simulink model "fsproje"  (R2023a)
settings: Solver=daessc  StartTime=0.0  StopTime=100  MaxStep=1e-2  RelTol=1e-3
values from neighbouring files (symbols this model uses):
  b = [0.01 1]    [tfsstwo.m]
  Kd = Kd + 10    (= 20)    [bessaniye.m]    (also in tfss.m = 0.25)
  Ki = 0    [bessaniye.m]    (also in tfss.m = 500)
  Kp = 100    [bessaniye.m]    (also in tfss.m = 21)
undefined symbols (not defined in the file or in its folder): B1, B2, J, J1, J2, K, K1, L, R
libraries: slpidlib x9
(part 1 of 2)
settings Model: Creator=monster  LastModifiedBy=monster
settings SolverCC: MaxConsecutiveMinStep=100000
settings DebuggingCC: MaskedZcDiagnostic=none  IgnoredZcDiagnostic=none

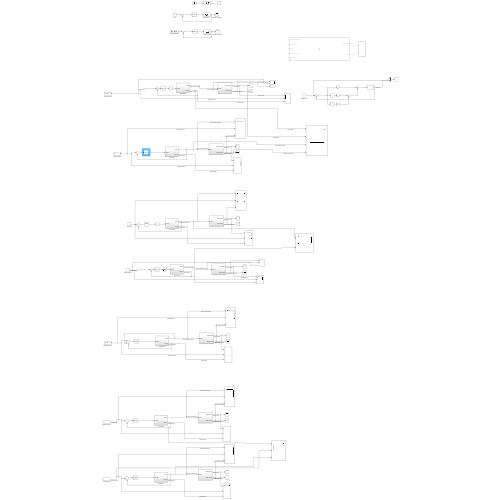
[thumbnail: Simulink's stored preview of the top-level diagram]
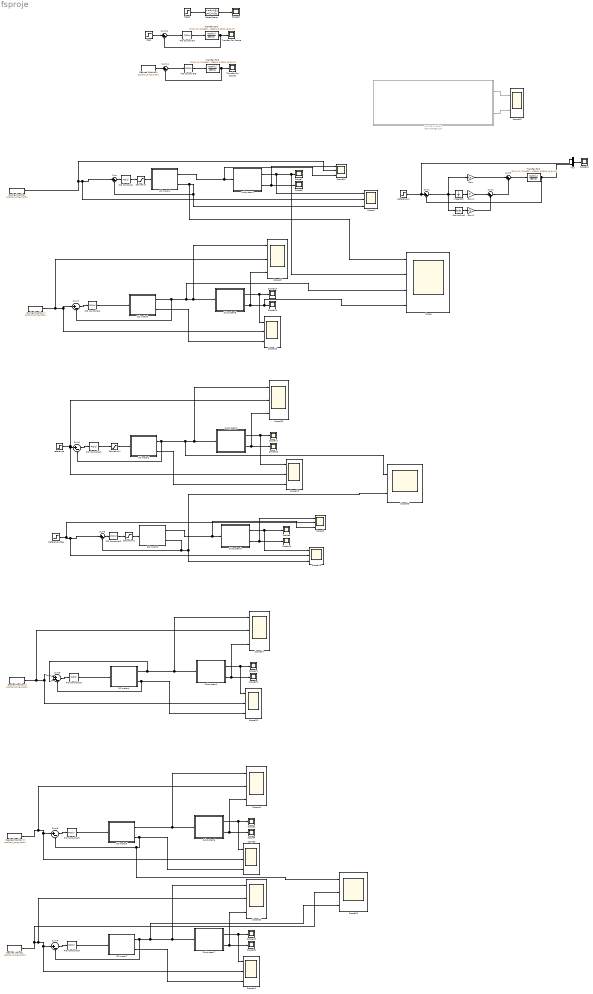
== system fsproje ==
  DC motor1 : Subsystem
  DC motor2 : Subsystem
  DC motor3 : Subsystem
  DC motor4 : Subsystem
  DC motor5 : Subsystem
  DC motor6 : Subsystem
  DC motor7 : Subsystem
  Derivative2 : Derivative
  Desired Position : FromWorkspace  VariableName=position_time_matrix
  Desired Position 1 : FromWorkspace  VariableName=position_time_matrix
  Desired Position 2 : FromWorkspace  VariableName=position_time_matrix
  Desired Position 3 : FromWorkspace  VariableName=position_time_matrix
  Desired Position1 : FromWorkspace  VariableName=position_time_matrix
  Desired Velocity : FromWorkspace  VariableName=position_time_matrix
  Gain : Gain  Gain=Kp
  Gain1 : Gain  Gain=Ki
  Gain2 : Gain  Gain=Kd
  Integrator : Integrator
  MATLAB Function : MATLAB Function  Commented=on  TreatAsAtomicUnit=on
  Mux : Mux  Inputs=2
  PID Controller : slpidlib/PID Controller  Controller=PID  Form=Parallel  TimeDomain=Continuous-time  UseExternalTs=off  SampleTime=-1  IntegratorMethod=Forward Euler  FilterMethod=Forward Euler  ControllerParametersSource=internal  P=58.5763414856901  I=21.7787994337213  UseKiTs=off  D=31.2977676191669  N=613.741127750797  UseFilter=on  TunerSelectOption=Transfer Function Based (PID Tuner App)  InitialConditionSource=internal  InitialConditionForIntegrator=0  InitialConditionForFilter=0  DifferentiatorICPrevScaledInput=0  ExternalReset=none  TrackingMode=off  Kt=1  LimitOutput=off  SatLimitsSource=internal  UpperSaturationLimit=10  LowerSaturationLimit=-10  LinearizeAsGain=on  AntiWindupMode=none  Kb=1  LimitIntegrator=off  UpperIntegratorSaturationLimit=10  LowerIntegratorSaturationLimit=-10  POutMin=[]  POutMax=[]  IOutMin=[]  IOutMax=[]  DOutMin=[]  DOutMax=[]  NOutMin=[]  NOutMax=[]  SumOutMin=[]  SumOutMax=[]  SaturationOutMin=[]  SaturationOutMax=[]  PParamMin=[]  PParamMax=[]  IParamMin=[]  IParamMax=[]  DParamMin=[]  DParamMax=[]  NParamMin=[]  NParamMax=[]  KbParamMin=[]  KbParamMax=[]  KtParamMin=[]  KtParamMax=[]  KbOutMin=[]  KbOutMax=[]  KtOutMin=[]  KtOutMax=[]  IntegratorOutMin=[]  IntegratorOutMax=[]  FilterOutMin=[]  FilterOutMax=[]  SumI1OutMin=[]  SumI1OutMax=[]  SumI2OutMin=[]  SumI2OutMax=[]  SumI3OutMin=[]  SumI3OutMax=[]  SumI4OutMin=[]  SumI4OutMax=[]  SumDOutMin=[]  SumDOutMax=[]  DifferentiatorOutMin=[]  DifferentiatorOutMax=[]  FilterDiffOutCoefMin=[]  FilterDiffOutCoefMax=[]  ReciprocalOutMin=[]  ReciprocalOutMax=[]  SumDenOutMin=[]  SumDenOutMax=[]  SumNumOutMin=[]  SumNumOutMax=[]  DivideOutMin=[]  DivideOutMax=[]  UdiffTsProdOutMin=[]  UdiffTsProdOutMax=[]  NTsProdOutMin=[]  NTsProdOutMax=[]  UintegralTsProdOutMin=[]  UintegralTsProdOutMax=[]  UngainTsProdOutMin=[]  UngainTsProdOutMax=[]  ClampingZeroOutDataTypeStr=Inherit: Inherit via back propagation  ClampingZeroOutMin=[]  ClampingZeroOutMax=[]  FilterDenConstantOutDataTypeStr=Inherit: Inherit via back propagation  FilterDenConstantOutMin=[]  FilterDenConstantOutMax=[]  PCopyOutDataTypeStr=Inherit: Inherit via back propagation  PCopyOutMin=[]  PCopyOutMax=[]  NCopyOutDataTypeStr=Inherit: Inherit via back propagation  NCopyOutMin=[]  NCopyOutMax=[]  IntegratorContinuousStateAttributes=''  IntegratorStateMustResolveToSignalObject=off  IntegratorRTWStateStorageClass=Auto  FilterContinuousStateAttributes=''  FilterStateMustResolveToSignalObject=off  FilterRTWStateStorageClass=Auto  ParallelPVariant=InternalParameters  IdealPVariant=Disabled  IVariant=InternalParameters  DVariant=InternalParameters  IntegratorVariant=Continuous  SatVariant=Disabled  AWVariant=Passthrough  PCopyVariant=Disabled  TRVariant=Disabled  FdbkBlocksVariant=Forward  IdealPFdbkVariant=Disabled  SatFdbkVariant=Disabled  DerivativeFilterVariant=ContFilter  NVariant=InternalParameters  NCopyVariant=Disabled  FilterICVariant=InternalICsFilter  IntegratorICVariant=InternalICs  ExternalResetVariant=Disabled  TRSumVariant=Passthrough  SumFdbkVariant=Disabled  SumVariant=Sum_PID  TsampFilterVariant=InternalTs  TsampNgainVariant=Passthrough  TsampIntegralVariant=Disabled_SignalSpec  ExternalSaturationOutDataTypeStr=Inherit: Same as second input
  PID Controller1 : slpidlib/PID Controller  Controller=PID  Form=Parallel  TimeDomain=Continuous-time  UseExternalTs=off  SampleTime=-1  IntegratorMethod=Forward Euler  FilterMethod=Forward Euler  ControllerParametersSource=internal  P=7.90320095450987  I=25.0422088343632  UseKiTs=off  D=0  N=100  UseFilter=on  TunerSelectOption=Transfer Function Based (PID Tuner App)  InitialConditionSource=internal  InitialConditionForIntegrator=0  InitialConditionForFilter=0  DifferentiatorICPrevScaledInput=0  ExternalReset=none  TrackingMode=off  Kt=1  LimitOutput=off  SatLimitsSource=internal  UpperSaturationLimit=10  LowerSaturationLimit=-10  LinearizeAsGain=on  AntiWindupMode=none  Kb=1  LimitIntegrator=off  UpperIntegratorSaturationLimit=10  LowerIntegratorSaturationLimit=-10  POutMin=[]  POutMax=[]  IOutMin=[]  IOutMax=[]  DOutMin=[]  DOutMax=[]  NOutMin=[]  NOutMax=[]  SumOutMin=[]  SumOutMax=[]  SaturationOutMin=[]  SaturationOutMax=[]  PParamMin=[]  PParamMax=[]  IParamMin=[]  IParamMax=[]  DParamMin=[]  DParamMax=[]  NParamMin=[]  NParamMax=[]  KbParamMin=[]  KbParamMax=[]  KtParamMin=[]  KtParamMax=[]  KbOutMin=[]  KbOutMax=[]  KtOutMin=[]  KtOutMax=[]  IntegratorOutMin=[]  IntegratorOutMax=[]  FilterOutMin=[]  FilterOutMax=[]  SumI1OutMin=[]  SumI1OutMax=[]  SumI2OutMin=[]  SumI2OutMax=[]  SumI3OutMin=[]  SumI3OutMax=[]  SumI4OutMin=[]  SumI4OutMax=[]  SumDOutMin=[]  SumDOutMax=[]  DifferentiatorOutMin=[]  DifferentiatorOutMax=[]  FilterDiffOutCoefMin=[]  FilterDiffOutCoefMax=[]  ReciprocalOutMin=[]  ReciprocalOutMax=[]  SumDenOutMin=[]  SumDenOutMax=[]  SumNumOutMin=[]  SumNumOutMax=[]  DivideOutMin=[]  DivideOutMax=[]  UdiffTsProdOutMin=[]  UdiffTsProdOutMax=[]  NTsProdOutMin=[]  NTsProdOutMax=[]  UintegralTsProdOutMin=[]  UintegralTsProdOutMax=[]  UngainTsProdOutMin=[]  UngainTsProdOutMax=[]  ClampingZeroOutDataTypeStr=Inherit: Inherit via back propagation  ClampingZeroOutMin=[]  ClampingZeroOutMax=[]  FilterDenConstantOutDataTypeStr=Inherit: Inherit via back propagation  FilterDenConstantOutMin=[]  FilterDenConstantOutMax=[]  PCopyOutDataTypeStr=Inherit: Inherit via back propagation  PCopyOutMin=[]  PCopyOutMax=[]  NCopyOutDataTypeStr=Inherit: Inherit via back propagation  NCopyOutMin=[]  NCopyOutMax=[]  IntegratorContinuousStateAttributes=''  IntegratorStateMustResolveToSignalObject=off  IntegratorRTWStateStorageClass=Auto  FilterContinuousStateAttributes=''  FilterStateMustResolveToSignalObject=off  FilterRTWStateStorageClass=Auto  ParallelPVariant=InternalParameters  IdealPVariant=Disabled  IVariant=InternalParameters  DVariant=InternalParameters  IntegratorVariant=Continuous  SatVariant=Disabled  AWVariant=Passthrough  PCopyVariant=Disabled  TRVariant=Disabled  FdbkBlocksVariant=Forward  IdealPFdbkVariant=Disabled  SatFdbkVariant=Disabled  DerivativeFilterVariant=ContFilter  NVariant=InternalParameters  NCopyVariant=Disabled  FilterICVariant=InternalICsFilter  IntegratorICVariant=InternalICs  ExternalResetVariant=Disabled  TRSumVariant=Passthrough  SumFdbkVariant=Disabled  SumVariant=Sum_PID  TsampFilterVariant=InternalTs  TsampNgainVariant=Passthrough  TsampIntegralVariant=Disabled_SignalSpec  ExternalSaturationOutDataTypeStr=Inherit: Same as second input
  PID Controller2 : slpidlib/PID Controller  Controller=PID  Form=Parallel  TimeDomain=Continuous-time  UseExternalTs=off  SampleTime=-1  IntegratorMethod=Forward Euler  FilterMethod=Forward Euler  ControllerParametersSource=internal  P=37.6557555770709  I=10.9348159465012  UseKiTs=off  D=22.0175242854137  N=444.616143119656  UseFilter=on  TunerSelectOption=Transfer Function Based (PID Tuner App)  InitialConditionSource=internal  InitialConditionForIntegrator=0  InitialConditionForFilter=0  DifferentiatorICPrevScaledInput=0  ExternalReset=none  TrackingMode=off  Kt=1  LimitOutput=off  SatLimitsSource=internal  UpperSaturationLimit=10  LowerSaturationLimit=-10  LinearizeAsGain=on  AntiWindupMode=none  Kb=1  LimitIntegrator=off  UpperIntegratorSaturationLimit=10  LowerIntegratorSaturationLimit=-10  POutMin=[]  POutMax=[]  IOutMin=[]  IOutMax=[]  DOutMin=[]  DOutMax=[]  NOutMin=[]  NOutMax=[]  SumOutMin=[]  SumOutMax=[]  SaturationOutMin=[]  SaturationOutMax=[]  PParamMin=[]  PParamMax=[]  IParamMin=[]  IParamMax=[]  DParamMin=[]  DParamMax=[]  NParamMin=[]  NParamMax=[]  KbParamMin=[]  KbParamMax=[]  KtParamMin=[]  KtParamMax=[]  KbOutMin=[]  KbOutMax=[]  KtOutMin=[]  KtOutMax=[]  IntegratorOutMin=[]  IntegratorOutMax=[]  FilterOutMin=[]  FilterOutMax=[]  SumI1OutMin=[]  SumI1OutMax=[]  SumI2OutMin=[]  SumI2OutMax=[]  SumI3OutMin=[]  SumI3OutMax=[]  SumI4OutMin=[]  SumI4OutMax=[]  SumDOutMin=[]  SumDOutMax=[]  DifferentiatorOutMin=[]  DifferentiatorOutMax=[]  FilterDiffOutCoefMin=[]  FilterDiffOutCoefMax=[]  ReciprocalOutMin=[]  ReciprocalOutMax=[]  SumDenOutMin=[]  SumDenOutMax=[]  SumNumOutMin=[]  SumNumOutMax=[]  DivideOutMin=[]  DivideOutMax=[]  UdiffTsProdOutMin=[]  UdiffTsProdOutMax=[]  NTsProdOutMin=[]  NTsProdOutMax=[]  UintegralTsProdOutMin=[]  UintegralTsProdOutMax=[]  UngainTsProdOutMin=[]  UngainTsProdOutMax=[]  ClampingZeroOutDataTypeStr=Inherit: Inherit via back propagation  ClampingZeroOutMin=[]  ClampingZeroOutMax=[]  FilterDenConstantOutDataTypeStr=Inherit: Inherit via back propagation  FilterDenConstantOutMin=[]  FilterDenConstantOutMax=[]  PCopyOutDataTypeStr=Inherit: Inherit via back propagation  PCopyOutMin=[]  PCopyOutMax=[]  NCopyOutDataTypeStr=Inherit: Inherit via back propagation  NCopyOutMin=[]  NCopyOutMax=[]  IntegratorContinuousStateAttributes=''  IntegratorStateMustResolveToSignalObject=off  IntegratorRTWStateStorageClass=Auto  FilterContinuousStateAttributes=''  FilterStateMustResolveToSignalObject=off  FilterRTWStateStorageClass=Auto  ParallelPVariant=InternalParameters  IdealPVariant=Disabled  IVariant=InternalParameters  DVariant=InternalParameters  IntegratorVariant=Continuous  SatVariant=Disabled  AWVariant=Passthrough  PCopyVariant=Disabled  TRVariant=Disabled  FdbkBlocksVariant=Forward  IdealPFdbkVariant=Disabled  SatFdbkVariant=Disabled  DerivativeFilterVariant=ContFilter  NVariant=InternalParameters  NCopyVariant=Disabled  FilterICVariant=InternalICsFilter  IntegratorICVariant=InternalICs  ExternalResetVariant=Disabled  TRSumVariant=Passthrough  SumFdbkVariant=Disabled  SumVariant=Sum_PID  TsampFilterVariant=InternalTs  TsampNgainVariant=Passthrough  TsampIntegralVariant=Disabled_SignalSpec  ExternalSaturationOutDataTypeStr=Inherit: Same as second input
  PID Controller3 : slpidlib/PID Controller  Controller=PID  Form=Parallel  TimeDomain=Continuous-time  UseExternalTs=off  SampleTime=-1  IntegratorMethod=Forward Euler  FilterMethod=Forward Euler  ControllerParametersSource=internal  P=2045.61485829821  I=4710.89336025682  UseKiTs=off  D=197.362863240612  N=45112.732739996  UseFilter=on  TunerSelectOption=Transfer Function Based (PID Tuner App)  InitialConditionSource=internal  InitialConditionForIntegrator=0  InitialConditionForFilter=0  DifferentiatorICPrevScaledInput=0  ExternalReset=none  TrackingMode=off  Kt=1  LimitOutput=off  SatLimitsSource=internal  UpperSaturationLimit=10  LowerSaturationLimit=-10  LinearizeAsGain=on  AntiWindupMode=none  Kb=1  LimitIntegrator=off  UpperIntegratorSaturationLimit=10  LowerIntegratorSaturationLimit=-10  POutMin=[]  POutMax=[]  IOutMin=[]  IOutMax=[]  DOutMin=[]  DOutMax=[]  NOutMin=[]  NOutMax=[]  SumOutMin=[]  SumOutMax=[]  SaturationOutMin=[]  SaturationOutMax=[]  PParamMin=[]  PParamMax=[]  IParamMin=[]  IParamMax=[]  DParamMin=[]  DParamMax=[]  NParamMin=[]  NParamMax=[]  KbParamMin=[]  KbParamMax=[]  KtParamMin=[]  KtParamMax=[]  KbOutMin=[]  KbOutMax=[]  KtOutMin=[]  KtOutMax=[]  IntegratorOutMin=[]  IntegratorOutMax=[]  FilterOutMin=[]  FilterOutMax=[]  SumI1OutMin=[]  SumI1OutMax=[]  SumI2OutMin=[]  SumI2OutMax=[]  SumI3OutMin=[]  SumI3OutMax=[]  SumI4OutMin=[]  SumI4OutMax=[]  SumDOutMin=[]  SumDOutMax=[]  DifferentiatorOutMin=[]  DifferentiatorOutMax=[]  FilterDiffOutCoefMin=[]  FilterDiffOutCoefMax=[]  ReciprocalOutMin=[]  ReciprocalOutMax=[]  SumDenOutMin=[]  SumDenOutMax=[]  SumNumOutMin=[]  SumNumOutMax=[]  DivideOutMin=[]  DivideOutMax=[]  UdiffTsProdOutMin=[]  UdiffTsProdOutMax=[]  NTsProdOutMin=[]  NTsProdOutMax=[]  UintegralTsProdOutMin=[]  UintegralTsProdOutMax=[]  UngainTsProdOutMin=[]  UngainTsProdOutMax=[]  ClampingZeroOutDataTypeStr=Inherit: Inherit via back propagation  ClampingZeroOutMin=[]  ClampingZeroOutMax=[]  FilterDenConstantOutDataTypeStr=Inherit: Inherit via back propagation  FilterDenConstantOutMin=[]  FilterDenConstantOutMax=[]  PCopyOutDataTypeStr=Inherit: Inherit via back propagation  PCopyOutMin=[]  PCopyOutMax=[]  NCopyOutDataTypeStr=Inherit: Inherit via back propagation  NCopyOutMin=[]  NCopyOutMax=[]  IntegratorContinuousStateAttributes=''  IntegratorStateMustResolveToSignalObject=off  IntegratorRTWStateStorageClass=Auto  FilterContinuousStateAttributes=''  FilterStateMustResolveToSignalObject=off  FilterRTWStateStorageClass=Auto  ParallelPVariant=InternalParameters  IdealPVariant=Disabled  IVariant=InternalParameters  DVariant=InternalParameters  IntegratorVariant=Continuous  SatVariant=Disabled  AWVariant=Passthrough  PCopyVariant=Disabled  TRVariant=Disabled  FdbkBlocksVariant=Forward  IdealPFdbkVariant=Disabled  SatFdbkVariant=Disabled  DerivativeFilterVariant=ContFilter  NVariant=InternalParameters  NCopyVariant=Disabled  FilterICVariant=InternalICsFilter  IntegratorICVariant=InternalICs  ExternalResetVariant=Disabled  TRSumVariant=Passthrough  SumFdbkVariant=Disabled  SumVariant=Sum_PID  TsampFilterVariant=InternalTs  TsampNgainVariant=Passthrough  TsampIntegralVariant=Disabled_SignalSpec  ExternalSaturationOutDataTypeStr=Inherit: Same as second input
  PID Controller4 : slpidlib/PID Controller  Controller=PID  Form=Parallel  TimeDomain=Continuous-time  UseExternalTs=off  SampleTime=-1  IntegratorMethod=Forward Euler  FilterMethod=Forward Euler  ControllerParametersSource=internal  P=207.324508460429  I=588.794544524933  UseKiTs=off  D=17.9277897178062  N=4054.94741877744  UseFilter=on  TunerSelectOption=Transfer Function Based (PID Tuner App)  InitialConditionSource=internal  InitialConditionForIntegrator=0  InitialConditionForFilter=0  DifferentiatorICPrevScaledInput=0  ExternalReset=none  TrackingMode=off  Kt=1  LimitOutput=off  SatLimitsSource=internal  UpperSaturationLimit=10  LowerSaturationLimit=-10  LinearizeAsGain=on  AntiWindupMode=none  Kb=1  LimitIntegrator=off  UpperIntegratorSaturationLimit=10  LowerIntegratorSaturationLimit=-10  POutMin=[]  POutMax=[]  IOutMin=[]  IOutMax=[]  DOutMin=[]  DOutMax=[]  NOutMin=[]  NOutMax=[]  SumOutMin=[]  SumOutMax=[]  SaturationOutMin=[]  SaturationOutMax=[]  PParamMin=[]  PParamMax=[]  IParamMin=[]  IParamMax=[]  DParamMin=[]  DParamMax=[]  NParamMin=[]  NParamMax=[]  KbParamMin=[]  KbParamMax=[]  KtParamMin=[]  KtParamMax=[]  KbOutMin=[]  KbOutMax=[]  KtOutMin=[]  KtOutMax=[]  IntegratorOutMin=[]  IntegratorOutMax=[]  FilterOutMin=[]  FilterOutMax=[]  SumI1OutMin=[]  SumI1OutMax=[]  SumI2OutMin=[]  SumI2OutMax=[]  SumI3OutMin=[]  SumI3OutMax=[]  SumI4OutMin=[]  SumI4OutMax=[]  SumDOutMin=[]  SumDOutMax=[]  DifferentiatorOutMin=[]  DifferentiatorOutMax=[]  FilterDiffOutCoefMin=[]  FilterDiffOutCoefMax=[]  ReciprocalOutMin=[]  ReciprocalOutMax=[]  SumDenOutMin=[]  SumDenOutMax=[]  SumNumOutMin=[]  SumNumOutMax=[]  DivideOutMin=[]  DivideOutMax=[]  UdiffTsProdOutMin=[]  UdiffTsProdOutMax=[]  NTsProdOutMin=[]  NTsProdOutMax=[]  UintegralTsProdOutMin=[]  UintegralTsProdOutMax=[]  UngainTsProdOutMin=[]  UngainTsProdOutMax=[]  ClampingZeroOutDataTypeStr=Inherit: Inherit via back propagation  ClampingZeroOutMin=[]  ClampingZeroOutMax=[]  FilterDenConstantOutDataTypeStr=Inherit: Inherit via back propagation  FilterDenConstantOutMin=[]  FilterDenConstantOutMax=[]  PCopyOutDataTypeStr=Inherit: Inherit via back propagation  PCopyOutMin=[]  PCopyOutMax=[]  NCopyOutDataTypeStr=Inherit: Inherit via back propagation  NCopyOutMin=[]  NCopyOutMax=[]  IntegratorContinuousStateAttributes=''  IntegratorStateMustResolveToSignalObject=off  IntegratorRTWStateStorageClass=Auto  FilterContinuousStateAttributes=''  FilterStateMustResolveToSignalObject=off  FilterRTWStateStorageClass=Auto  ParallelPVariant=InternalParameters  IdealPVariant=Disabled  IVariant=InternalParameters  DVariant=InternalParameters  IntegratorVariant=Continuous  SatVariant=Disabled  AWVariant=Passthrough  PCopyVariant=Disabled  TRVariant=Disabled  FdbkBlocksVariant=Forward  IdealPFdbkVariant=Disabled  SatFdbkVariant=Disabled  DerivativeFilterVariant=ContFilter  NVariant=InternalParameters  NCopyVariant=Disabled  FilterICVariant=InternalICsFilter  IntegratorICVariant=InternalICs  ExternalResetVariant=Disabled  TRSumVariant=Passthrough  SumFdbkVariant=Disabled  SumVariant=Sum_PID  TsampFilterVariant=InternalTs  TsampNgainVariant=Passthrough  TsampIntegralVariant=Disabled_SignalSpec  ExternalSaturationOutDataTypeStr=Inherit: Same as second input
  PID Controller5 : slpidlib/PID Controller  Controller=PID  Form=Parallel  TimeDomain=Continuous-time  UseExternalTs=off  SampleTime=-1  IntegratorMethod=Forward Euler  FilterMethod=Forward Euler  ControllerParametersSource=internal  P=55.9637536976089  I=20.0064460537914  UseKiTs=off  D=29.6071796486486  N=586.118226738446  UseFilter=on  TunerSelectOption=Transfer Function Based (PID Tuner App)  InitialConditionSource=internal  InitialConditionForIntegrator=0  InitialConditionForFilter=0  DifferentiatorICPrevScaledInput=0  ExternalReset=none  TrackingMode=off  Kt=1  LimitOutput=off  SatLimitsSource=internal  UpperSaturationLimit=10  LowerSaturationLimit=-10  LinearizeAsGain=on  AntiWindupMode=none  Kb=1  LimitIntegrator=off  UpperIntegratorSaturationLimit=10  LowerIntegratorSaturationLimit=-10  POutMin=[]  POutMax=[]  IOutMin=[]  IOutMax=[]  DOutMin=[]  DOutMax=[]  NOutMin=[]  NOutMax=[]  SumOutMin=[]  SumOutMax=[]  SaturationOutMin=[]  SaturationOutMax=[]  PParamMin=[]  PParamMax=[]  IParamMin=[]  IParamMax=[]  DParamMin=[]  DParamMax=[]  NParamMin=[]  NParamMax=[]  KbParamMin=[]  KbParamMax=[]  KtParamMin=[]  KtParamMax=[]  KbOutMin=[]  KbOutMax=[]  KtOutMin=[]  KtOutMax=[]  IntegratorOutMin=[]  IntegratorOutMax=[]  FilterOutMin=[]  FilterOutMax=[]  SumI1OutMin=[]  SumI1OutMax=[]  SumI2OutMin=[]  SumI2OutMax=[]  SumI3OutMin=[]  SumI3OutMax=[]  SumI4OutMin=[]  SumI4OutMax=[]  SumDOutMin=[]  SumDOutMax=[]  DifferentiatorOutMin=[]  DifferentiatorOutMax=[]  FilterDiffOutCoefMin=[]  FilterDiffOutCoefMax=[]  ReciprocalOutMin=[]  ReciprocalOutMax=[]  SumDenOutMin=[]  SumDenOutMax=[]  SumNumOutMin=[]  SumNumOutMax=[]  DivideOutMin=[]  DivideOutMax=[]  UdiffTsProdOutMin=[]  UdiffTsProdOutMax=[]  NTsProdOutMin=[]  NTsProdOutMax=[]  UintegralTsProdOutMin=[]  UintegralTsProdOutMax=[]  UngainTsProdOutMin=[]  UngainTsProdOutMax=[]  ClampingZeroOutDataTypeStr=Inherit: Inherit via back propagation  ClampingZeroOutMin=[]  ClampingZeroOutMax=[]  FilterDenConstantOutDataTypeStr=Inherit: Inherit via back propagation  FilterDenConstantOutMin=[]  FilterDenConstantOutMax=[]  PCopyOutDataTypeStr=Inherit: Inherit via back propagation  PCopyOutMin=[]  PCopyOutMax=[]  NCopyOutDataTypeStr=Inherit: Inherit via back propagation  NCopyOutMin=[]  NCopyOutMax=[]  IntegratorContinuousStateAttributes=''  IntegratorStateMustResolveToSignalObject=off  IntegratorRTWStateStorageClass=Auto  FilterContinuousStateAttributes=''  FilterStateMustResolveToSignalObject=off  FilterRTWStateStorageClass=Auto  ParallelPVariant=InternalParameters  IdealPVariant=Disabled  IVariant=InternalParameters  DVariant=InternalParameters  IntegratorVariant=Continuous  SatVariant=Disabled  AWVariant=Passthrough  PCopyVariant=Disabled  TRVariant=Disabled  FdbkBlocksVariant=Forward  IdealPFdbkVariant=Disabled  SatFdbkVariant=Disabled  DerivativeFilterVariant=ContFilter  NVariant=InternalParameters  NCopyVariant=Disabled  FilterICVariant=InternalICsFilter  IntegratorICVariant=InternalICs  ExternalResetVariant=Disabled  TRSumVariant=Passthrough  SumFdbkVariant=Disabled  SumVariant=Sum_PID  TsampFilterVariant=InternalTs  TsampNgainVariant=Passthrough  TsampIntegralVariant=Disabled_SignalSpec  ExternalSaturationOutDataTypeStr=Inherit: Same as second input
  PID Controller6 : slpidlib/PID Controller  Controller=PID  Form=Parallel  TimeDomain=Continuous-time  UseExternalTs=off  SampleTime=-1  IntegratorMethod=Forward Euler  FilterMethod=Forward Euler  ControllerParametersSource=internal  P=18.2217269934491  I=51.328469994586  UseKiTs=off  D=0.957542307400605  N=37.219289351236  UseFilter=on  TunerSelectOption=Transfer Function Based (PID Tuner App)  InitialConditionSource=internal  InitialConditionForIntegrator=0  InitialConditionForFilter=0  DifferentiatorICPrevScaledInput=0  ExternalReset=none  TrackingMode=off  Kt=1  LimitOutput=off  SatLimitsSource=internal  UpperSaturationLimit=10  LowerSaturationLimit=-10  LinearizeAsGain=on  AntiWindupMode=none  Kb=1  LimitIntegrator=off  UpperIntegratorSaturationLimit=10  LowerIntegratorSaturationLimit=-10  POutMin=[]  POutMax=[]  IOutMin=[]  IOutMax=[]  DOutMin=[]  DOutMax=[]  NOutMin=[]  NOutMax=[]  SumOutMin=[]  SumOutMax=[]  SaturationOutMin=[]  SaturationOutMax=[]  PParamMin=[]  PParamMax=[]  IParamMin=[]  IParamMax=[]  DParamMin=[]  DParamMax=[]  NParamMin=[]  NParamMax=[]  KbParamMin=[]  KbParamMax=[]  KtParamMin=[]  KtParamMax=[]  KbOutMin=[]  KbOutMax=[]  KtOutMin=[]  KtOutMax=[]  IntegratorOutMin=[]  IntegratorOutMax=[]  FilterOutMin=[]  FilterOutMax=[]  SumI1OutMin=[]  SumI1OutMax=[]  SumI2OutMin=[]  SumI2OutMax=[]  SumI3OutMin=[]  SumI3OutMax=[]  SumI4OutMin=[]  SumI4OutMax=[]  SumDOutMin=[]  SumDOutMax=[]  DifferentiatorOutMin=[]  DifferentiatorOutMax=[]  FilterDiffOutCoefMin=[]  FilterDiffOutCoefMax=[]  ReciprocalOutMin=[]  ReciprocalOutMax=[]  SumDenOutMin=[]  SumDenOutMax=[]  SumNumOutMin=[]  SumNumOutMax=[]  DivideOutMin=[]  DivideOutMax=[]  UdiffTsProdOutMin=[]  UdiffTsProdOutMax=[]  NTsProdOutMin=[]  NTsProdOutMax=[]  UintegralTsProdOutMin=[]  UintegralTsProdOutMax=[]  UngainTsProdOutMin=[]  UngainTsProdOutMax=[]  ClampingZeroOutDataTypeStr=Inherit: Inherit via back propagation  ClampingZeroOutMin=[]  ClampingZeroOutMax=[]  FilterDenConstantOutDataTypeStr=Inherit: Inherit via back propagation  FilterDenConstantOutMin=[]  FilterDenConstantOutMax=[]  PCopyOutDataTypeStr=Inherit: Inherit via back propagation  PCopyOutMin=[]  PCopyOutMax=[]  NCopyOutDataTypeStr=Inherit: Inherit via back propagation  NCopyOutMin=[]  NCopyOutMax=[]  IntegratorContinuousStateAttributes=''  IntegratorStateMustResolveToSignalObject=off  IntegratorRTWStateStorageClass=Auto  FilterContinuousStateAttributes=''  FilterStateMustResolveToSignalObject=off  FilterRTWStateStorageClass=Auto  ParallelPVariant=InternalParameters  IdealPVariant=Disabled  IVariant=InternalParameters  DVariant=InternalParameters  IntegratorVariant=Continuous  SatVariant=Disabled  AWVariant=Passthrough  PCopyVariant=Disabled  TRVariant=Disabled  FdbkBlocksVariant=Forward  IdealPFdbkVariant=Disabled  SatFdbkVariant=Disabled  DerivativeFilterVariant=ContFilter  NVariant=InternalParameters  NCopyVariant=Disabled  FilterICVariant=InternalICsFilter  IntegratorICVariant=InternalICs  ExternalResetVariant=Disabled  TRSumVariant=Passthrough  SumFdbkVariant=Disabled  SumVariant=Sum_PID  TsampFilterVariant=InternalTs  TsampNgainVariant=Passthrough  TsampIntegralVariant=Disabled_SignalSpec  ExternalSaturationOutDataTypeStr=Inherit: Same as second input
  PID Controller7 : slpidlib/PID Controller  Controller=PID  Form=Parallel  TimeDomain=Continuous-time  UseExternalTs=off  SampleTime=-1  IntegratorMethod=Forward Euler  FilterMethod=Forward Euler  ControllerParametersSource=internal  P=40.9250284632695  I=11.6471169726926  UseKiTs=off  D=18.6506512361338  N=402.948949977405  UseFilter=on  TunerSelectOption=Transfer Function Based (PID Tuner App)  InitialConditionSource=internal  InitialConditionForIntegrator=0  InitialConditionForFilter=0  DifferentiatorICPrevScaledInput=0  ExternalReset=none  TrackingMode=off  Kt=1  LimitOutput=off  SatLimitsSource=internal  UpperSaturationLimit=inf  LowerSaturationLimit=-inf  LinearizeAsGain=on  AntiWindupMode=none  Kb=1  LimitIntegrator=off  UpperIntegratorSaturationLimit=inf  LowerIntegratorSaturationLimit=-inf  POutMin=[]  POutMax=[]  IOutMin=[]  IOutMax=[]  DOutMin=[]  DOutMax=[]  NOutMin=[]  NOutMax=[]  SumOutMin=[]  SumOutMax=[]  SaturationOutMin=[]  SaturationOutMax=[]  PParamMin=[]  PParamMax=[]  IParamMin=[]  IParamMax=[]  DParamMin=[]  DParamMax=[]  NParamMin=[]  NParamMax=[]  KbParamMin=[]  KbParamMax=[]  KtParamMin=[]  KtParamMax=[]  KbOutMin=[]  KbOutMax=[]  KtOutMin=[]  KtOutMax=[]  IntegratorOutMin=[]  IntegratorOutMax=[]  FilterOutMin=[]  FilterOutMax=[]  SumI1OutMin=[]  SumI1OutMax=[]  SumI2OutMin=[]  SumI2OutMax=[]  SumI3OutMin=[]  SumI3OutMax=[]  SumI4OutMin=[]  SumI4OutMax=[]  SumDOutMin=[]  SumDOutMax=[]  DifferentiatorOutMin=[]  DifferentiatorOutMax=[]  FilterDiffOutCoefMin=[]  FilterDiffOutCoefMax=[]  ReciprocalOutMin=[]  ReciprocalOutMax=[]  SumDenOutMin=[]  SumDenOutMax=[]  SumNumOutMin=[]  SumNumOutMax=[]  DivideOutMin=[]  DivideOutMax=[]  UdiffTsProdOutMin=[]  UdiffTsProdOutMax=[]  NTsProdOutMin=[]  NTsProdOutMax=[]  UintegralTsProdOutMin=[]  UintegralTsProdOutMax=[]  UngainTsProdOutMin=[]  UngainTsProdOutMax=[]  ClampingZeroOutDataTypeStr=Inherit: Inherit via back propagation  ClampingZeroOutMin=[]  ClampingZeroOutMax=[]  FilterDenConstantOutDataTypeStr=Inherit: Inherit via back propagation  FilterDenConstantOutMin=[]  FilterDenConstantOutMax=[]  PCopyOutDataTypeStr=Inherit: Inherit via back propagation  PCopyOutMin=[]  PCopyOutMax=[]  NCopyOutDataTypeStr=Inherit: Inherit via back propagation  NCopyOutMin=[]  NCopyOutMax=[]  IntegratorContinuousStateAttributes=''  IntegratorStateMustResolveToSignalObject=off  IntegratorRTWStateStorageClass=Auto  FilterContinuousStateAttributes=''  FilterStateMustResolveToSignalObject=off  FilterRTWStateStorageClass=Auto  ParallelPVariant=InternalParameters  IdealPVariant=Disabled  IVariant=InternalParameters  DVariant=InternalParameters  IntegratorVariant=Continuous  SatVariant=Disabled  AWVariant=Passthrough  PCopyVariant=Disabled  TRVariant=Disabled  FdbkBlocksVariant=Forward  IdealPFdbkVariant=Disabled  SatFdbkVariant=Disabled  DerivativeFilterVariant=ContFilter  NVariant=InternalParameters  NCopyVariant=Disabled  FilterICVariant=InternalICsFilter  IntegratorICVariant=InternalICs  ExternalResetVariant=Disabled  TRSumVariant=Passthrough  SumFdbkVariant=Disabled  SumVariant=Sum_PID  TsampFilterVariant=InternalTs  TsampNgainVariant=Passthrough  TsampIntegralVariant=Disabled_SignalSpec  ExternalSaturationOutDataTypeStr=Inherit: Same as second input
  PID Controller8 : slpidlib/PID Controller  Controller=PID  Form=Parallel  TimeDomain=Continuous-time  UseExternalTs=off  SampleTime=-1  IntegratorMethod=Forward Euler  FilterMethod=Forward Euler  ControllerParametersSource=internal  P=40.9250284632695  I=11.6471169726926  UseKiTs=off  D=18.6506512361338  N=402.948949977405  UseFilter=on  TunerSelectOption=Transfer Function Based (PID Tuner App)  InitialConditionSource=internal  InitialConditionForIntegrator=0  InitialConditionForFilter=0  DifferentiatorICPrevScaledInput=0  ExternalReset=none  TrackingMode=off  Kt=1  LimitOutput=off  SatLimitsSource=internal  UpperSaturationLimit=inf  LowerSaturationLimit=-inf  LinearizeAsGain=on  AntiWindupMode=none  Kb=1  LimitIntegrator=off  UpperIntegratorSaturationLimit=inf  LowerIntegratorSaturationLimit=-inf  POutMin=[]  POutMax=[]  IOutMin=[]  IOutMax=[]  DOutMin=[]  DOutMax=[]  NOutMin=[]  NOutMax=[]  SumOutMin=[]  SumOutMax=[]  SaturationOutMin=[]  SaturationOutMax=[]  PParamMin=[]  PParamMax=[]  IParamMin=[]  IParamMax=[]  DParamMin=[]  DParamMax=[]  NParamMin=[]  NParamMax=[]  KbParamMin=[]  KbParamMax=[]  KtParamMin=[]  KtParamMax=[]  KbOutMin=[]  KbOutMax=[]  KtOutMin=[]  KtOutMax=[]  IntegratorOutMin=[]  IntegratorOutMax=[]  FilterOutMin=[]  FilterOutMax=[]  SumI1OutMin=[]  SumI1OutMax=[]  SumI2OutMin=[]  SumI2OutMax=[]  SumI3OutMin=[]  SumI3OutMax=[]  SumI4OutMin=[]  SumI4OutMax=[]  SumDOutMin=[]  SumDOutMax=[]  DifferentiatorOutMin=[]  DifferentiatorOutMax=[]  FilterDiffOutCoefMin=[]  FilterDiffOutCoefMax=[]  ReciprocalOutMin=[]  ReciprocalOutMax=[]  SumDenOutMin=[]  SumDenOutMax=[]  SumNumOutMin=[]  SumNumOutMax=[]  DivideOutMin=[]  DivideOutMax=[]  UdiffTsProdOutMin=[]  UdiffTsProdOutMax=[]  NTsProdOutMin=[]  NTsProdOutMax=[]  UintegralTsProdOutMin=[]  UintegralTsProdOutMax=[]  UngainTsProdOutMin=[]  UngainTsProdOutMax=[]  ClampingZeroOutDataTypeStr=Inherit: Inherit via back propagation  ClampingZeroOutMin=[]  ClampingZeroOutMax=[]  FilterDenConstantOutDataTypeStr=Inherit: Inherit via back propagation  FilterDenConstantOutMin=[]  FilterDenConstantOutMax=[]  PCopyOutDataTypeStr=Inherit: Inherit via back propagation  PCopyOutMin=[]  PCopyOutMax=[]  NCopyOutDataTypeStr=Inherit: Inherit via back propagation  NCopyOutMin=[]  NCopyOutMax=[]  IntegratorContinuousStateAttributes=''  IntegratorStateMustResolveToSignalObject=off  IntegratorRTWStateStorageClass=Auto  FilterContinuousStateAttributes=''  FilterStateMustResolveToSignalObject=off  FilterRTWStateStorageClass=Auto  ParallelPVariant=InternalParameters  IdealPVariant=Disabled  IVariant=InternalParameters  DVariant=InternalParameters  IntegratorVariant=Continuous  SatVariant=Disabled  AWVariant=Passthrough  PCopyVariant=Disabled  TRVariant=Disabled  FdbkBlocksVariant=Forward  IdealPFdbkVariant=Disabled  SatFdbkVariant=Disabled  DerivativeFilterVariant=ContFilter  NVariant=InternalParameters  NCopyVariant=Disabled  FilterICVariant=InternalICsFilter  IntegratorICVariant=InternalICs  ExternalResetVariant=Disabled  TRSumVariant=Passthrough  SumFdbkVariant=Disabled  SumVariant=Sum_PID  TsampFilterVariant=InternalTs  TsampNgainVariant=Passthrough  TsampIntegralVariant=Disabled_SignalSpec  ExternalSaturationOutDataTypeStr=Inherit: Same as second input
  Reference 2 : Step  SampleTime=0
  Reference Step : Step  After=5  SampleTime=0
  Saturation : Saturate  UpperLimit=50  LowerLimit=-50
  Saturation1 : Saturate  UpperLimit=100000  LowerLimit=-100000
  Saturation2 : Saturate  UpperLimit=100000  LowerLimit=-100000
  Scope : Scope  NumInputPorts=4
  Scope{1,3,9..10,13..14,19..20,23..24,26..28,31..32} (15 alike) : Scope  NumInputPorts=3
  Scope{2,4..8,11..12,15,17..18,21..22,25,29..30} (16 alike) : Scope
  Scope16 : Scope  NumInputPorts=2
  Scope33 : Scope  NumInputPorts=2
  State-Space : StateSpace  A=[-32 -1260 -12400 -20020 0; 1 0 0 0 0; 0 1 0 0 0; 0 0 1 0 0; 0 0 0 1 0]  B=[1; 0; 0; 0; 0]  C=[0 0 0 20 2000]  D=[0]  InitialCondition=[0;0;0;0;0]
  Step : Step  After=5  SampleTime=0
  Step2 : Step  After=5  SampleTime=0
  Subsystem1 : Subsystem
  Subsystem2 : Subsystem
  Subsystem3 : Subsystem
  Subsystem4 : Subsystem
  Subsystem5 : Subsystem
  Subsystem6 : Subsystem
  Subsystem7 : Subsystem
  Sum{,1,4..5,7..11} (9 alike) : Sum  Inputs=|+-
  Sum2 : Sum  Inputs=|++
  Sum3 : Sum  Inputs=|++
  Sum6 : Sum  Inputs=|+--
  Transfer Fcn Scope : Scope
  Transfer Fcn Scope1 : Scope
  Transfer Fcn1 : TransferFcn  Numerator=[0.01 1]  Denominator=[0.0005 0.016 0.63001 6.2002 10.01 0]
  Transfer Fcn2 : TransferFcn  Numerator=[0.01 1]  Denominator=[0.0005 0.016 0.63001 6.2002 10.01 0]
  Transfer Fcn3 : TransferFcn  Numerator=[0.01 1]  Denominator=[0.0005 0.016 0.63001 6.2002 10.01 0]
  reference : Step  After=5  SampleTime=0
  wires:
  Integrator/1 -> Gain1/1
  DC motor2/1(Speed) -> Scope33/1, Scope20/1, Subsystem2/1(Speed), Sum4/2  "Motor Velocity Simulink"
  Gain1/1 -> Sum2/1
  MATLAB Function/1(position_radian) -> Scope16/1
  reference/1 -> Sum4/1, Scope19/2, Scope20/2
  Sum/1 -> PID Controller/1
  Reference 2/1 -> Mux/1, Sum1/1
  Sum4/1 -> PID Controller1/1
  Subsystem2/2(Shaft Velocity) -> Scope20/3, Scope18/1  "Shaft Velocity Simulink"
  Gain/1 -> Sum3/1
  Transfer Fcn2/1 -> Sum1/2, Mux/2  "Position"
  Subsystem1/2(Shaft Velocity) -> Scope10/1, Scope8/1  "Shaft Velocity Simulink"
  MATLAB Function/2(velocity) -> Scope16/2
  Saturation/1 -> DC motor1/1(voltage)
  Subsystem1/1(Shaft Position) -> Scope1/1, Scope/2, Scope7/1  "Shaft Position"
  Gain2/1 -> Sum2/2
  Sum2/1 -> Sum3/2
  Derivative2/1 -> Gain2/1
  Subsystem2/1(Shaft Position) -> Scope19/1, Scope17/1  "Shaft Position"
  PID Controller/1 -> Saturation/1
  Sum3/1 -> Transfer Fcn2/1
  Sum1/1 -> Derivative2/1, Gain/1, Integrator/1
  DC motor2/2(Position) -> Scope19/3  "Motor Position"
  DC motor1/1(Speed) -> Scope10/3, Subsystem1/1(Speed)  "Motor Velocity Simulink"
  Mux/1 -> Scope12/1
  PID Controller1/1 -> Saturation1/1
  DC motor1/2(Position) -> Scope/1, Scope1/3, Sum/2  "Motor Position"
  State-Space/1 -> Scope5/1
  Step2/1 -> State-Space/1
  Transfer Fcn1/1 -> Transfer Fcn Scope/1, Sum10/2
  Desired Position/1 -> Scope10/2, Scope1/2, Sum/1  "Desired Position"
  Saturation1/1 -> DC motor2/1(voltage)
  Reference Step/1 -> Scope13/2, Sum5/1, Scope3/2  "Reference step"
  DC motor3/2(Position) -> Sum5/2, Scope33/2, Scope13/3  "Motor Position"
  PID Controller2/1 -> Saturation2/1
  DC motor3/1(Speed) -> Scope3/3, Subsystem3/1(Speed)  "Motor Velocity Simulink"
  Subsystem3/1(Shaft Position) -> Scope13/1, Scope6/1  "Shaft Position"
  Subsystem3/2(Shaft Velocity) -> Scope3/1, Scope11/1  "Shaft Velocity Simulink"
  Saturation2/1 -> DC motor3/1(voltage)
  Sum5/1 -> PID Controller2/1
  Subsystem4/2(Shaft Velocity) -> Scope24/3, Scope22/1  "Shaft Velocity Simulink"
  Sum6/1 -> PID Controller3/1
  DC motor4/2(Position) -> Scope23/3, Sum6/3  "Motor Position"
  Subsystem4/1(Shaft Position) -> Scope23/1, Scope21/1  "Shaft Position"
  DC motor4/1(Speed) -> Sum6/2, Scope24/1, Subsystem4/1(Speed)  "Motor Velocity Simulink"
  Desired Position 2/1 -> Scope24/2, Scope23/2, Sum6/1  "Desired Position 2"
  PID Controller3/1 -> DC motor4/1(voltage)
  DC motor5/2(Position) -> Scope26/3  "Motor Position"
  Desired Position 1/1 -> Scope27/2, Scope26/2, Sum7/1  "Desired Position 2"
  PID Controller4/1 -> DC motor5/1(voltage)
  Sum7/1 -> PID Controller4/1
  Subsystem5/2(Shaft Velocity) -> Scope27/3, Scope/4, Scope25/1  "Shaft Velocity Simulink"
  DC motor5/1(Speed) -> Scope/3, Scope27/1, Subsystem5/1(Speed), Sum7/2  "Motor Velocity Simulink"
  Subsystem5/1(Shaft Position) -> Scope26/1, Scope15/1  "Shaft Position"
  PID Controller5/1 -> DC motor6/1(voltage)
  DC motor6/2(Position) -> Scope32/1, Sum8/2, Scope9/3  "Motor Position"
  DC motor6/1(Speed) -> Scope14/1, Subsystem6/1(Speed)  "Motor Velocity Simulink"
  Subsystem6/1(Shaft Position) -> Scope9/1, Scope2/1  "Shaft Position"
  Subsystem6/2(Shaft Velocity) -> Scope14/3, Scope4/1  "Shaft Velocity Simulink"
  Sum8/1 -> PID Controller5/1
  Desired Position 3/1 -> Scope14/2, Scope9/2, Sum8/1  "Desired Position"
  Desired Velocity/1 -> Scope32/2, Sum9/1, Scope31/2, Scope28/2  "Desired Velocity"
  Sum9/1 -> PID Controller6/1
  Subsystem7/2(Shaft Velocity) -> Scope30/1, Scope28/3  "Shaft Velocity Simulink"
  Subsystem7/1(Shaft Position) -> Scope29/1, Scope31/1  "Shaft Position"
  DC motor7/1(Speed) -> Scope32/3, Subsystem7/1(Speed), Scope28/1, Sum9/2  "Motor Velocity Simulink"
  DC motor7/2(Position) -> Scope31/3  "Motor Position"
  PID Controller6/1 -> DC motor7/1(voltage)
  PID Controller7/1 -> Transfer Fcn1/1
  Step/1 -> Sum10/1
  Sum10/1 -> PID Controller7/1
  PID Controller8/1 -> Transfer Fcn3/1
  Transfer Fcn3/1 -> Transfer Fcn Scope1/1, Sum11/2
  Sum11/1 -> PID Controller8/1
  Desired Position1/1 -> Sum11/1

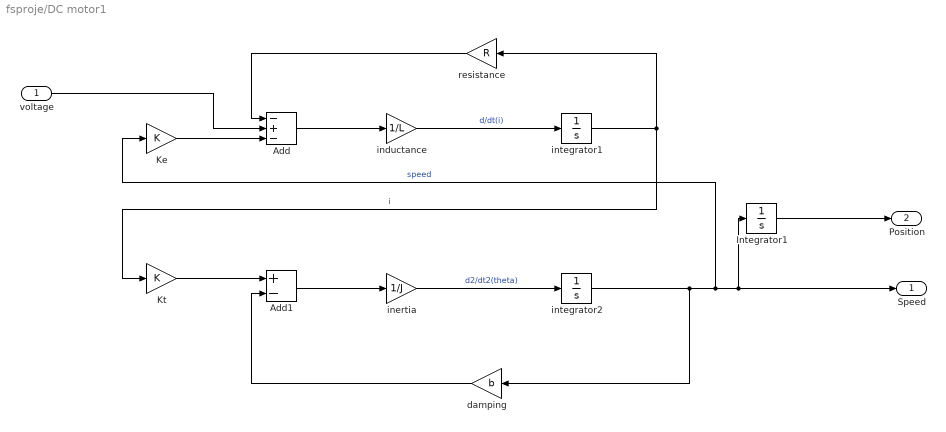
== system fsproje/DC motor1 ==
  voltage : Inport
  Add : Sum  Inputs=-+-
  Add1 : Sum  Inputs=+-
  Integrator1 : Integrator
  Ke : Gain  Gain=K
  Kt : Gain  Gain=K
  damping : Gain  Gain=b
  "inductance " : Gain  Gain=1/L
  inertia : Gain  Gain=1/J
  integrator1 : Integrator
  integrator2 : Integrator
  resistance : Gain  Gain=R
  Speed : Outport
  Position : Outport  Port=2
  wires:
  damping/1 -> Add1/2
  Add1/1 -> inertia/1
  Kt/1 -> Add1/1
  integrator1/1 -> resistance/1, Kt/1  "i"
  Add/1 -> "inductance "/1
  voltage/1 -> Add/2
  resistance/1 -> Add/1
  inertia/1 -> integrator2/1  "d2/dt2(theta)"
  integrator2/1 -> damping/1, Integrator1/1, Speed/1, Ke/1  "speed"
  Ke/1 -> Add/3
  "inductance "/1 -> integrator1/1  "d/dt(i)"
  Integrator1/1 -> Position/1

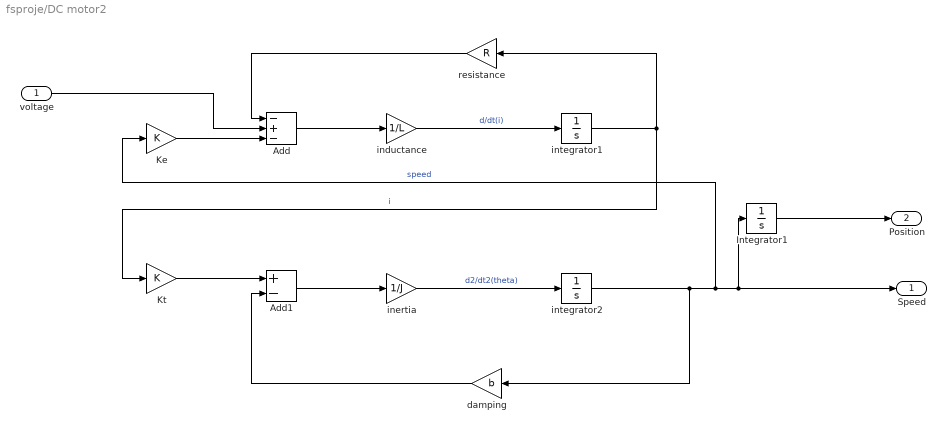
== system fsproje/DC motor2 ==
  voltage : Inport
  Add : Sum  Inputs=-+-
  Add1 : Sum  Inputs=+-
  Integrator1 : Integrator
  Ke : Gain  Gain=K
  Kt : Gain  Gain=K
  damping : Gain  Gain=b
  "inductance " : Gain  Gain=1/L
  inertia : Gain  Gain=1/J
  integrator1 : Integrator
  integrator2 : Integrator
  resistance : Gain  Gain=R
  Speed : Outport
  Position : Outport  Port=2
  wires:
  damping/1 -> Add1/2
  Add1/1 -> inertia/1
  Kt/1 -> Add1/1
  integrator1/1 -> resistance/1, Kt/1  "i"
  Add/1 -> "inductance "/1
  voltage/1 -> Add/2
  resistance/1 -> Add/1
  inertia/1 -> integrator2/1  "d2/dt2(theta)"
  integrator2/1 -> damping/1, Integrator1/1, Speed/1, Ke/1  "speed"
  Ke/1 -> Add/3
  "inductance "/1 -> integrator1/1  "d/dt(i)"
  Integrator1/1 -> Position/1

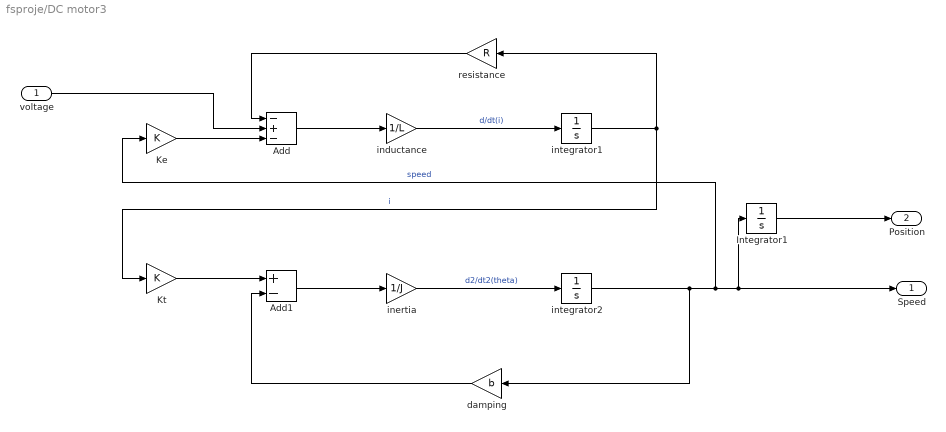
== system fsproje/DC motor3 ==
  voltage : Inport
  Add : Sum  Inputs=-+-
  Add1 : Sum  Inputs=+-
  Integrator1 : Integrator
  Ke : Gain  Gain=K
  Kt : Gain  Gain=K
  damping : Gain  Gain=b
  "inductance " : Gain  Gain=1/L
  inertia : Gain  Gain=1/J
  integrator1 : Integrator
  integrator2 : Integrator
  resistance : Gain  Gain=R
  Speed : Outport
  Position : Outport  Port=2
  wires:
  damping/1 -> Add1/2
  Add1/1 -> inertia/1
  Kt/1 -> Add1/1
  integrator1/1 -> resistance/1, Kt/1  "i"
  Add/1 -> "inductance "/1
  voltage/1 -> Add/2
  resistance/1 -> Add/1
  inertia/1 -> integrator2/1  "d2/dt2(theta)"
  integrator2/1 -> damping/1, Integrator1/1, Speed/1, Ke/1  "speed"
  Ke/1 -> Add/3
  "inductance "/1 -> integrator1/1  "d/dt(i)"
  Integrator1/1 -> Position/1

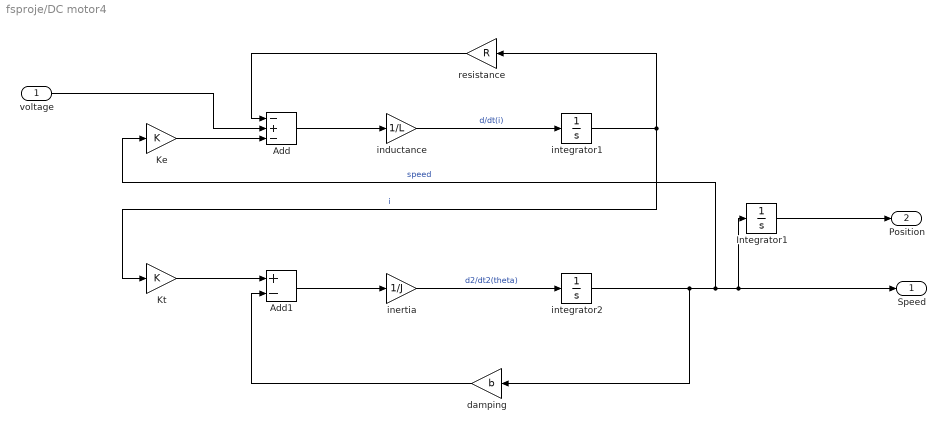
== system fsproje/DC motor4 ==
  voltage : Inport
  Add : Sum  Inputs=-+-
  Add1 : Sum  Inputs=+-
  Integrator1 : Integrator
  Ke : Gain  Gain=K
  Kt : Gain  Gain=K
  damping : Gain  Gain=b
  "inductance " : Gain  Gain=1/L
  inertia : Gain  Gain=1/J
  integrator1 : Integrator
  integrator2 : Integrator
  resistance : Gain  Gain=R
  Speed : Outport
  Position : Outport  Port=2
  wires:
  damping/1 -> Add1/2
  Add1/1 -> inertia/1
  Kt/1 -> Add1/1
  integrator1/1 -> resistance/1, Kt/1  "i"
  Add/1 -> "inductance "/1
  voltage/1 -> Add/2
  resistance/1 -> Add/1
  inertia/1 -> integrator2/1  "d2/dt2(theta)"
  integrator2/1 -> damping/1, Integrator1/1, Speed/1, Ke/1  "speed"
  Ke/1 -> Add/3
  "inductance "/1 -> integrator1/1  "d/dt(i)"
  Integrator1/1 -> Position/1

== system fsproje/DC motor5 ==
  voltage : Inport
  Add : Sum  Inputs=-+-
  Add1 : Sum  Inputs=+-
  Integrator1 : Integrator
  Ke : Gain  Gain=K
  Kt : Gain  Gain=K
  damping : Gain  Gain=b
  "inductance " : Gain  Gain=1/L
  inertia : Gain  Gain=1/J
  integrator1 : Integrator
  integrator2 : Integrator
  resistance : Gain  Gain=R
  Speed : Outport
  Position : Outport  Port=2
  wires:
  damping/1 -> Add1/2
  Add1/1 -> inertia/1
  Kt/1 -> Add1/1
  integrator1/1 -> resistance/1, Kt/1  "i"
  Add/1 -> "inductance "/1
  voltage/1 -> Add/2
  resistance/1 -> Add/1
  inertia/1 -> integrator2/1  "d2/dt2(theta)"
  integrator2/1 -> damping/1, Integrator1/1, Speed/1, Ke/1  "speed"
  Ke/1 -> Add/3
  "inductance "/1 -> integrator1/1  "d/dt(i)"
  Integrator1/1 -> Position/1

== system fsproje/DC motor6 ==
  voltage : Inport
  Add : Sum  Inputs=-+-
  Add1 : Sum  Inputs=+-
  Integrator1 : Integrator
  Ke : Gain  Gain=K
  Kt : Gain  Gain=K
  damping : Gain  Gain=b
  "inductance " : Gain  Gain=1/L
  inertia : Gain  Gain=1/J
  integrator1 : Integrator
  integrator2 : Integrator
  resistance : Gain  Gain=R
  Speed : Outport
  Position : Outport  Port=2
  wires:
  damping/1 -> Add1/2
  Add1/1 -> inertia/1
  Kt/1 -> Add1/1
  integrator1/1 -> resistance/1, Kt/1  "i"
  Add/1 -> "inductance "/1
  voltage/1 -> Add/2
  resistance/1 -> Add/1
  inertia/1 -> integrator2/1  "d2/dt2(theta)"
  integrator2/1 -> damping/1, Integrator1/1, Speed/1, Ke/1  "speed"
  Ke/1 -> Add/3
  "inductance "/1 -> integrator1/1  "d/dt(i)"
  Integrator1/1 -> Position/1

== system fsproje/DC motor7 ==
  voltage : Inport
  Add : Sum  Inputs=-+-
  Add1 : Sum  Inputs=+-
  Integrator1 : Integrator
  Ke : Gain  Gain=K
  Kt : Gain  Gain=K
  damping : Gain  Gain=b
  "inductance " : Gain  Gain=1/L
  inertia : Gain  Gain=1/J
  integrator1 : Integrator
  integrator2 : Integrator
  resistance : Gain  Gain=R
  Speed : Outport
  Position : Outport  Port=2
  wires:
  Integrator1/1 -> Position/1
  "inductance "/1 -> integrator1/1  "d/dt(i)"
  Ke/1 -> Add/3
  integrator2/1 -> Ke/1, Speed/1, Integrator1/1, damping/1  "speed"
  inertia/1 -> integrator2/1  "d2/dt2(theta)"
  resistance/1 -> Add/1
  voltage/1 -> Add/2
  Add/1 -> "inductance "/1
  integrator1/1 -> Kt/1, resistance/1  "i"
  Kt/1 -> Add1/1
  Add1/1 -> inertia/1
  damping/1 -> Add1/2

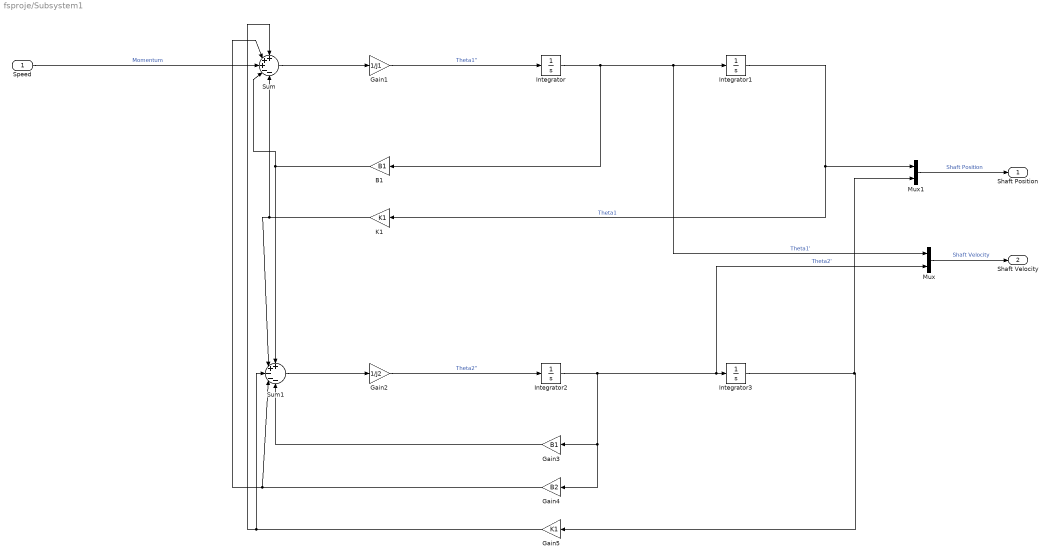
== system fsproje/Subsystem1 ==
  Speed : Inport
  B1 : Gain  Gain=B1
  Gain1 : Gain  Gain=1/J1
  Gain2 : Gain  Gain=1/J2
  Gain3 : Gain  Gain=B1
  Gain4 : Gain  Gain=B2
  Gain5 : Gain  Gain=K1
  Integrator{,1..3} (4 alike) : Integrator
  K1 : Gain  Gain=K1
  Mux : Mux  Inputs=2
  Mux1 : Mux  Inputs=2
  Sum : Sum  Inputs=+++--
  Sum1 : Sum  Inputs=++---
  Shaft Position : Outport
  Shaft Velocity : Outport  Port=2
  wires:
  Gain5/1 -> Sum1/3, Sum/1
  Integrator3/1 -> Gain5/1, Mux1/2
  Gain4/1 -> Sum/2, Sum1/4
  Gain3/1 -> Sum1/5
  Integrator2/1 -> Mux/2, Integrator3/1, Gain3/1, Gain4/1  "Theta2'"
  Gain2/1 -> Integrator2/1  "Theta2''"
  Sum1/1 -> Gain2/1
  K1/1 -> Sum1/2, Sum/5
  Integrator1/1 -> Mux1/1, K1/1  "Theta1"
  B1/1 -> Sum/4, Sum1/1
  Integrator/1 -> Mux/1, Integrator1/1, B1/1  "Theta1'"
  Gain1/1 -> Integrator/1  "Theta1''"
  Speed/1 -> Sum/3  "Momentum"
  Sum/1 -> Gain1/1
  Mux1/1 -> Shaft Position/1  "Shaft Position"
  Mux/1 -> Shaft Velocity/1  "Shaft Velocity"

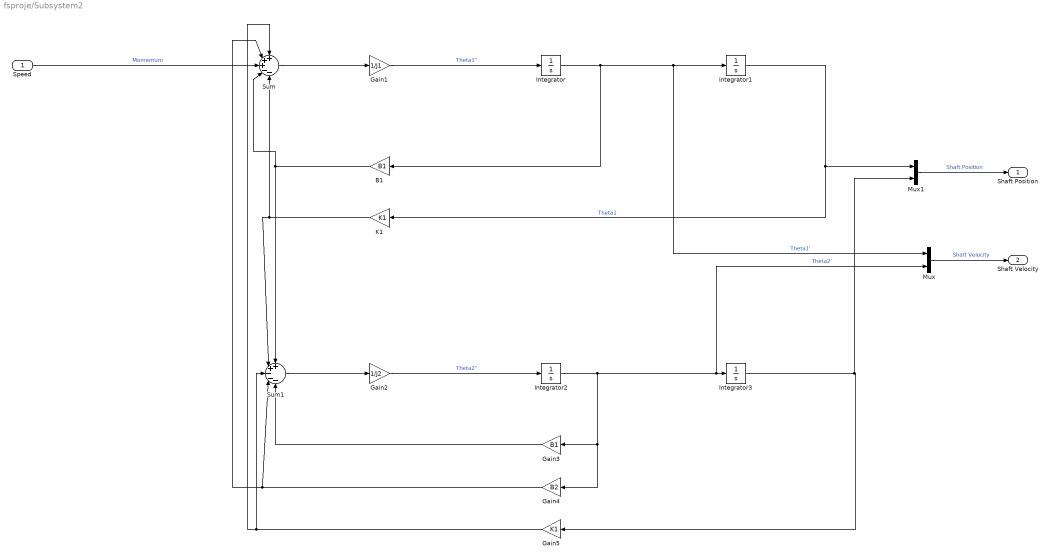
== system fsproje/Subsystem2 ==
  Speed : Inport
  B1 : Gain  Gain=B1
  Gain1 : Gain  Gain=1/J1
  Gain2 : Gain  Gain=1/J2
  Gain3 : Gain  Gain=B1
  Gain4 : Gain  Gain=B2
  Gain5 : Gain  Gain=K1
  Integrator{,1..3} (4 alike) : Integrator
  K1 : Gain  Gain=K1
  Mux : Mux  Inputs=2
  Mux1 : Mux  Inputs=2
  Sum : Sum  Inputs=+++--
  Sum1 : Sum  Inputs=++---
  Shaft Position : Outport
  Shaft Velocity : Outport  Port=2
  wires:
  Gain5/1 -> Sum1/3, Sum/1
  Integrator3/1 -> Gain5/1, Mux1/2
  Gain4/1 -> Sum/2, Sum1/4
  Gain3/1 -> Sum1/5
  Integrator2/1 -> Mux/2, Integrator3/1, Gain3/1, Gain4/1  "Theta2'"
  Gain2/1 -> Integrator2/1  "Theta2''"
  Sum1/1 -> Gain2/1
  K1/1 -> Sum1/2, Sum/5
  Integrator1/1 -> Mux1/1, K1/1  "Theta1"
  B1/1 -> Sum/4, Sum1/1
  Integrator/1 -> Mux/1, Integrator1/1, B1/1  "Theta1'"
  Gain1/1 -> Integrator/1  "Theta1''"
  Speed/1 -> Sum/3  "Momentum"
  Sum/1 -> Gain1/1
  Mux1/1 -> Shaft Position/1  "Shaft Position"
  Mux/1 -> Shaft Velocity/1  "Shaft Velocity"

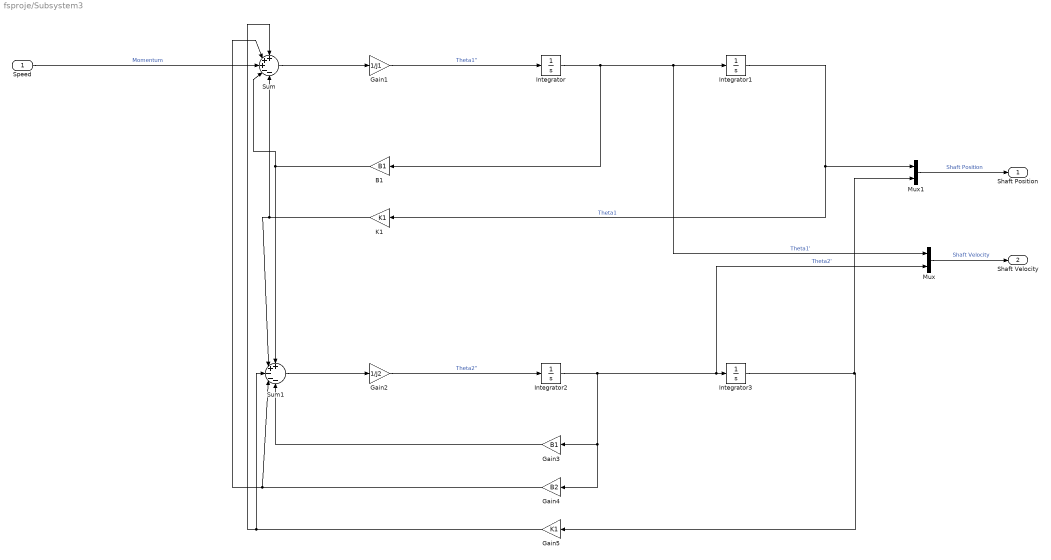
== system fsproje/Subsystem3 ==
  Speed : Inport
  B1 : Gain  Gain=B1
  Gain1 : Gain  Gain=1/J1
  Gain2 : Gain  Gain=1/J2
  Gain3 : Gain  Gain=B1
  Gain4 : Gain  Gain=B2
  Gain5 : Gain  Gain=K1
  Integrator{,1..3} (4 alike) : Integrator
  K1 : Gain  Gain=K1
  Mux : Mux  Inputs=2
  Mux1 : Mux  Inputs=2
  Sum : Sum  Inputs=+++--
  Sum1 : Sum  Inputs=++---
  Shaft Position : Outport
  Shaft Velocity : Outport  Port=2
  wires:
  Gain5/1 -> Sum1/3, Sum/1
  Integrator3/1 -> Gain5/1, Mux1/2
  Gain4/1 -> Sum/2, Sum1/4
  Gain3/1 -> Sum1/5
  Integrator2/1 -> Mux/2, Integrator3/1, Gain3/1, Gain4/1  "Theta2'"
  Gain2/1 -> Integrator2/1  "Theta2''"
  Sum1/1 -> Gain2/1
  K1/1 -> Sum1/2, Sum/5
  Integrator1/1 -> Mux1/1, K1/1  "Theta1"
  B1/1 -> Sum/4, Sum1/1
  Integrator/1 -> Mux/1, Integrator1/1, B1/1  "Theta1'"
  Gain1/1 -> Integrator/1  "Theta1''"
  Speed/1 -> Sum/3  "Momentum"
  Sum/1 -> Gain1/1
  Mux1/1 -> Shaft Position/1  "Shaft Position"
  Mux/1 -> Shaft Velocity/1  "Shaft Velocity"

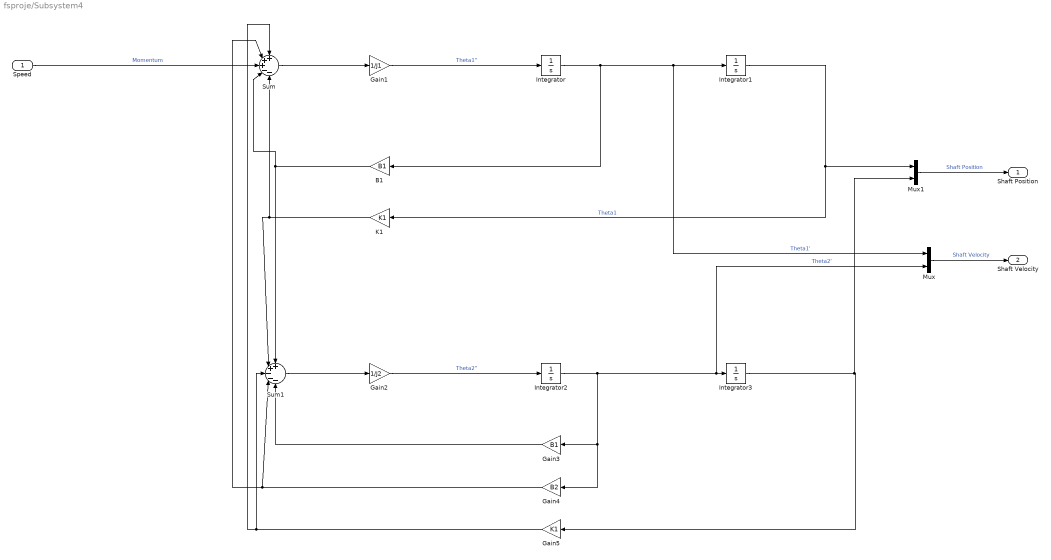
== system fsproje/Subsystem4 ==
  Speed : Inport
  B1 : Gain  Gain=B1
  Gain1 : Gain  Gain=1/J1
  Gain2 : Gain  Gain=1/J2
  Gain3 : Gain  Gain=B1
  Gain4 : Gain  Gain=B2
  Gain5 : Gain  Gain=K1
  Integrator{,1..3} (4 alike) : Integrator
  K1 : Gain  Gain=K1
  Mux : Mux  Inputs=2
  Mux1 : Mux  Inputs=2
  Sum : Sum  Inputs=+++--
  Sum1 : Sum  Inputs=++---
  Shaft Position : Outport
  Shaft Velocity : Outport  Port=2
  wires:
  Gain5/1 -> Sum1/3, Sum/1
  Integrator3/1 -> Gain5/1, Mux1/2
  Gain4/1 -> Sum/2, Sum1/4
  Gain3/1 -> Sum1/5
  Integrator2/1 -> Mux/2, Integrator3/1, Gain3/1, Gain4/1  "Theta2'"
  Gain2/1 -> Integrator2/1  "Theta2''"
  Sum1/1 -> Gain2/1
  K1/1 -> Sum1/2, Sum/5
  Integrator1/1 -> Mux1/1, K1/1  "Theta1"
  B1/1 -> Sum/4, Sum1/1
  Integrator/1 -> Mux/1, Integrator1/1, B1/1  "Theta1'"
  Gain1/1 -> Integrator/1  "Theta1''"
  Speed/1 -> Sum/3  "Momentum"
  Sum/1 -> Gain1/1
  Mux1/1 -> Shaft Position/1  "Shaft Position"
  Mux/1 -> Shaft Velocity/1  "Shaft Velocity"

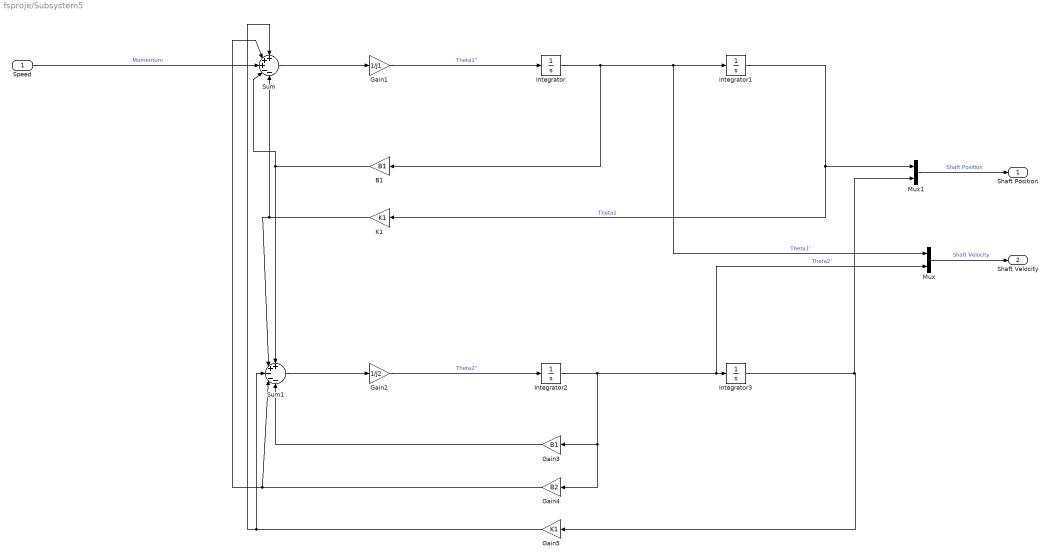
== system fsproje/Subsystem5 ==
  Speed : Inport
  B1 : Gain  Gain=B1
  Gain1 : Gain  Gain=1/J1
  Gain2 : Gain  Gain=1/J2
  Gain3 : Gain  Gain=B1
  Gain4 : Gain  Gain=B2
  Gain5 : Gain  Gain=K1
  Integrator{,1..3} (4 alike) : Integrator
  K1 : Gain  Gain=K1
  Mux : Mux  Inputs=2
  Mux1 : Mux  Inputs=2
  Sum : Sum  Inputs=+++--
  Sum1 : Sum  Inputs=++---
  Shaft Position : Outport
  Shaft Velocity : Outport  Port=2
  wires:
  Gain5/1 -> Sum1/3, Sum/1
  Integrator3/1 -> Gain5/1, Mux1/2
  Gain4/1 -> Sum/2, Sum1/4
  Gain3/1 -> Sum1/5
  Integrator2/1 -> Mux/2, Integrator3/1, Gain3/1, Gain4/1  "Theta2'"
  Gain2/1 -> Integrator2/1  "Theta2''"
  Sum1/1 -> Gain2/1
  K1/1 -> Sum1/2, Sum/5
  Integrator1/1 -> Mux1/1, K1/1  "Theta1"
  B1/1 -> Sum/4, Sum1/1
  Integrator/1 -> Mux/1, Integrator1/1, B1/1  "Theta1'"
  Gain1/1 -> Integrator/1  "Theta1''"
  Speed/1 -> Sum/3  "Momentum"
  Sum/1 -> Gain1/1
  Mux1/1 -> Shaft Position/1  "Shaft Position"
  Mux/1 -> Shaft Velocity/1  "Shaft Velocity"

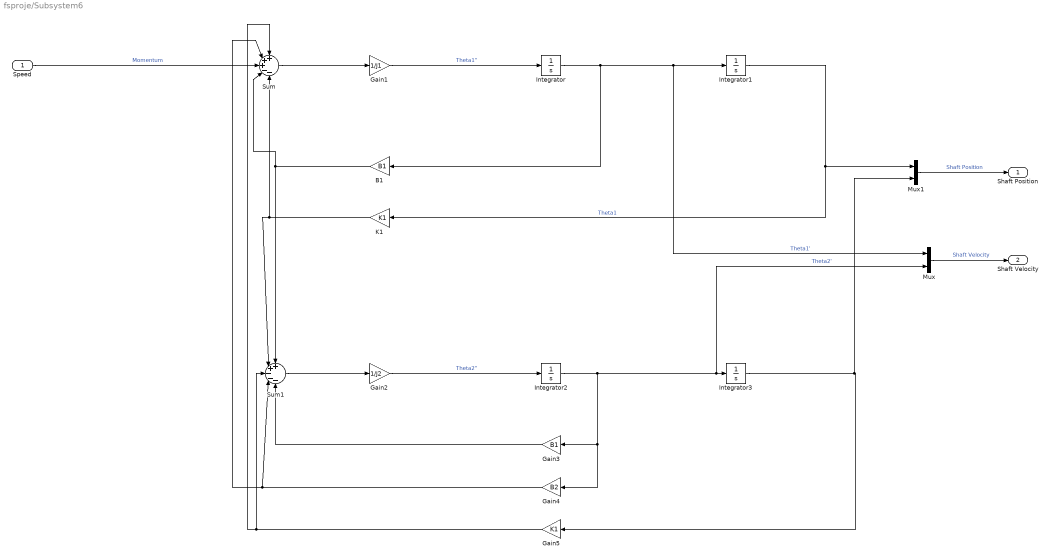
== system fsproje/Subsystem6 ==
  Speed : Inport
  B1 : Gain  Gain=B1
  Gain1 : Gain  Gain=1/J1
  Gain2 : Gain  Gain=1/J2
  Gain3 : Gain  Gain=B1
  Gain4 : Gain  Gain=B2
  Gain5 : Gain  Gain=K1
  Integrator{,1..3} (4 alike) : Integrator
  K1 : Gain  Gain=K1
  Mux : Mux  Inputs=2
  Mux1 : Mux  Inputs=2
  Sum : Sum  Inputs=+++--
  Sum1 : Sum  Inputs=++---
  Shaft Position : Outport
  Shaft Velocity : Outport  Port=2
  wires:
  Gain5/1 -> Sum1/3, Sum/1
  Integrator3/1 -> Gain5/1, Mux1/2
  Gain4/1 -> Sum/2, Sum1/4
  Gain3/1 -> Sum1/5
  Integrator2/1 -> Mux/2, Integrator3/1, Gain3/1, Gain4/1  "Theta2'"
  Gain2/1 -> Integrator2/1  "Theta2''"
  Sum1/1 -> Gain2/1
  K1/1 -> Sum1/2, Sum/5
  Integrator1/1 -> Mux1/1, K1/1  "Theta1"
  B1/1 -> Sum/4, Sum1/1
  Integrator/1 -> Mux/1, Integrator1/1, B1/1  "Theta1'"
  Gain1/1 -> Integrator/1  "Theta1''"
  Speed/1 -> Sum/3  "Momentum"
  Sum/1 -> Gain1/1
  Mux1/1 -> Shaft Position/1  "Shaft Position"
  Mux/1 -> Shaft Velocity/1  "Shaft Velocity"

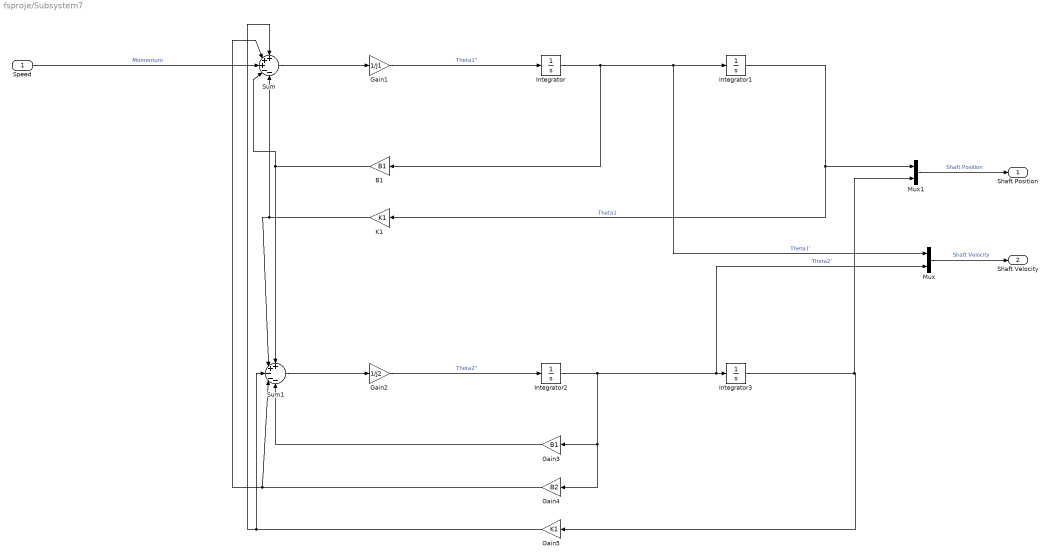
== system fsproje/Subsystem7 ==
  Speed : Inport
  B1 : Gain  Gain=B1
  Gain1 : Gain  Gain=1/J1
  Gain2 : Gain  Gain=1/J2
  Gain3 : Gain  Gain=B1
  Gain4 : Gain  Gain=B2
  Gain5 : Gain  Gain=K1
  Integrator{,1..3} (4 alike) : Integrator
  K1 : Gain  Gain=K1
  Mux : Mux  Inputs=2
  Mux1 : Mux  Inputs=2
  Sum : Sum  Inputs=+++--
  Sum1 : Sum  Inputs=++---
  Shaft Position : Outport
  Shaft Velocity : Outport  Port=2
  wires:
  Mux/1 -> Shaft Velocity/1  "Shaft Velocity"
  Mux1/1 -> Shaft Position/1  "Shaft Position"
  Sum/1 -> Gain1/1
  Speed/1 -> Sum/3  "Momentum"
  Gain1/1 -> Integrator/1  "Theta1''"
  Integrator/1 -> B1/1, Integrator1/1, Mux/1  "Theta1'"
  B1/1 -> Sum1/1, Sum/4
  Integrator1/1 -> K1/1, Mux1/1  "Theta1"
  K1/1 -> Sum/5, Sum1/2
  Sum1/1 -> Gain2/1
  Gain2/1 -> Integrator2/1  "Theta2''"
  Integrator2/1 -> Gain4/1, Gain3/1, Integrator3/1, Mux/2  "Theta2'"
  Gain3/1 -> Sum1/5
  Gain4/1 -> Sum1/4, Sum/2
  Integrator3/1 -> Mux1/2, Gain5/1
  Gain5/1 -> Sum/1, Sum1/3
